simulink model "LAB3_Challenge_SSM_LQR_FS"  (R2020b)
settings: Solver=ode45  StartTime=0.0  StopTime=Time_of_simulation  RelTol=1e-3
undefined symbols (not defined in the file): Aq, Bb, Beq, Bq, daq, denH_w, DiscIntNeverNeededParam, drv, enable_integrator, gbox, Jb, Jh, K, K_I, Kaw, mld, mot, Nu, numH_w, Nxa, rads2rpm, sens, Step_ref, tausf, Ts
libraries: simulink x4
settings Model: Creator=Davide  LastModifiedBy=Musta

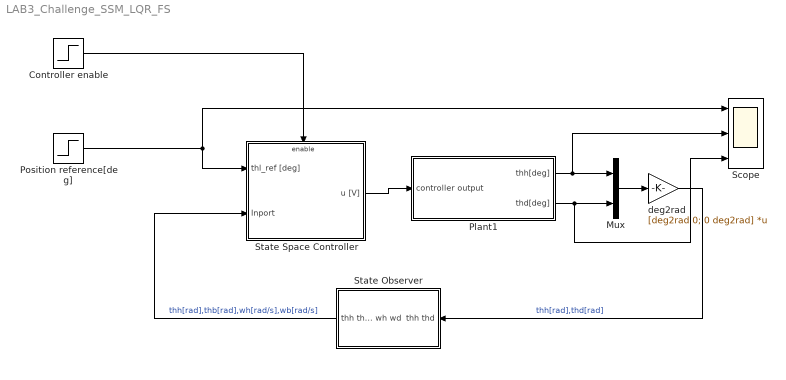
== system LAB3_Challenge_SSM_LQR_FS ==
  Controller enable : Step  Time=0.75  SampleTime=0
  Mux : Mux  Inputs=2
  Plant1 : Subsystem
  Position reference[deg] : Step  After=Step_ref  SampleTime=0
  Scope : Scope  NumInputPorts=3
  State Observer : Subsystem
  State Space Controller : Subsystem
  deg2rad : Gain  Gain=[deg2rad 0; 0 deg2rad]  Multiplication=Matrix(K*u) (u vector)
  wires:
  Position reference[deg]/1 -> Scope/1, State Space Controller/1(thl_ref [deg])
  Controller enable/1 -> State Space Controller/Enable
  Plant1/1(thh[deg]) -> Scope/2, Mux/1
  Mux/1 -> deg2rad/1
  deg2rad/1 -> State Observer/1(thh thd)  "thh[rad],thd[rad]"
  State Space Controller/1(u [V]) -> Plant1/1(controller output)
  Plant1/2(thd[deg]) -> Scope/3, Mux/2
  State Observer/1(thh thd wh wd) -> State Space Controller/2(Inport)  "thh[rad],thb[rad],wh[rad/s],wb[rad/s]"

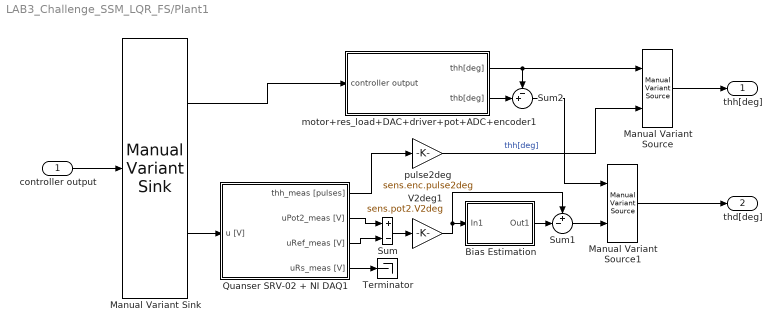
== system LAB3_Challenge_SSM_LQR_FS/Plant1 ==
  controller output : Inport
  Bias Estimation : Subsystem
  Manual Variant Sink : simulink/Signal Routing/Manual Variant Sink  NumChoices=2  LabelModeActiveChoice=V_2
  Manual Variant Source : simulink/Signal Routing/Manual Variant Source  NumChoices=2  LabelModeActiveChoice=V_2
  Manual Variant Source1 : simulink/Signal Routing/Manual Variant Source  NumChoices=2  LabelModeActiveChoice=V_2
  Quanser SRV-02 + NI DAQ1 : Subsystem  mask(Quanser SRV-02 (with resonant load) + NI DAQ){Ts=0.001, fricType=Karnopp, lockShaft=off, beamInitPos=10}
      mask prompts: Ts "NI DAQ Sample Time:"; fricType "Friction model"; lockShaft "Lock motor shaft"; beamInitPos "Beam initial position [deg]:"
      mask help: Quanser SRV-02 (with resonant load) + NI DAQ model.
      mask init:
      | %%
      | % Riccardo Antonello (riccardo.antonello@unipd.it)
      | %
      | % April 28, 2020
      | %
      | % Dept. of Information Engineering, University of Padova
      | %
      | 
      | %%  Conversion gains
      | deg2rad = pi/180;                   %   [deg]   -> [rad]
      | rad2deg = 180/pi;                   %   [rad]   -> [deg]
      | 
      | 
      | %%  Sensors data
      | 
      | %   shunt resistor
      | sens.curr.Rs = 0.5;   
      | 
      | %   Hewlett-Packard HEDS-5540#A06 optical encoder
      | sens.enc.ppr = 500*4;                                                   %   pulses per rotation
      | sens.enc.pulse2deg = 360/sens.enc.ppr;                                  %   [pulses] -> [deg]
      | sens.enc.pulse2rad = 2*pi/sens.enc.ppr;                                 %   [pulses] -> [rad]
      | sens.enc.deg2pulse = sens.enc.ppr/360;                                  %   [deg] -> [pulses]
      | sens.enc.rad2pulse = sens.enc.ppr/2/pi;                                 %   [rad] -> [pulses]
      | 
      | %   potentiometer 2 (Spectrol 357-0-0-103) - installed on hub
      | sens.pot2.range.R      = 10e3;                                          %   ohmic value range 
      | sens.pot2.range.V      = 5;                                             %   voltage range
      | sens.pot2.range.th_deg = 340;                                           %   angle range [deg]
      | sens.pot2.range.th     = sens.pot2.range.th_deg * deg2rad;              %   angle range [rad]                           
      | sens.pot2.deg2V        = sens.pot2.range.V / sens.pot2.range.th_deg;    %   sensitivity [V/deg]
      | sens.pot2.rad2V        = sens.pot2.range.V / sens.pot2.range.th;        %   sensitivity [V/rad]
      | sens.pot2.V2deg        = 1/sens.pot2.deg2V;                             %   conversion gain [V] -> [deg]
      | sens.pot2.V2rad        = 1/sens.pot2.rad2V;                             %   conversion gain [V] -> [rad]
      | sens.pot2.noise.var    = 3.5e-7;                                        %   out noise variance [V^2]
      | 
      | 
      | %%  Data acquisition board (daq) data
      | 
      | %   NI PCI-6221 DAC data
      | daq.dac.bits = 16;                                  %   resolution (bits)
      | daq.dac.fs   = 10;                                  %   full scale 
      | daq.dac.q    = 2*daq.dac.fs/(2^daq.dac.bits-1);     %	quantization
      | 
      | %   NI PCI-6221 ADC data
      | daq.adc.bits = 16;                                  %   resolution (bits)
      | daq.adc.fs   = 10;                                  %   full scale (as set in SLDRT Analog Input block)
      | daq.adc.q    = 2*daq.adc.fs/(2^daq.adc.bits-1);     %   quantization   
      | 
      | 
      | %%  Set beam initial position
      | % SRV02Handle = find_system(gcb, ...
      | %     'LookUnderMasks', 'on', ...
      | %     'FindAll', 'on', ...
      | %     'FollowLinks', 'on', ...
      | %     'SearchDepth', '1', ...
      | %     'BlockType', 'ModelReference', ...
      | %     'Name', 'Quanser SRV-02');
      | %
      | % %get_param(SRV02Handle, 'InstanceParameters')
      | % InstanceParams = get_param(SRV02Handle, 'InstanceParameters');
      | % for k = 1:length(InstanceParams)
      | %     if strcmp(InstanceParams(k).Name, 'thb0')
      | %         if lockShaft
      | %             InstanceParams(k).Value = sprintf('%f', beamInitPos);
      | %         else
      | %             InstanceParams(k).Value = sprintf('%f', 0);    
      | %         end
      | %         set_param(SRV02Handle, 'InstanceParameters', InstanceParams);
      | %         break;
      | %     end
      | % end
      | 
      | if lockShaft
      |     thb0 = beamInitPos;
      | else
      |     thb0 = 0;    
      | end
      | 
      | 
      | %%  Mask initialization
      | if lockShaft
      |     
      |     %   find Inport handle
      |     InPortHandle = find_system(gcb, ...
      |         'LookUnderMasks', 'on', ...
      |         'FindAll', 'on', ...
      |         'FollowLinks', 'on', ...
      |         'SearchDepth', '1', ...
      |         'BlockType', 'Inport', ...
      |         'Name', 'u [V]');
      |     
      |     if ~isempty(InPortHandle)
      |     
      |         %   find DAC handle
      |         DACHandle = find_system(gcb, ...
      |             'LookUnderMasks', 'on', ...
      |             'FindAll', 'on', ...
      |             'FollowLinks', 'on', ...
      |             'SearchDepth', '1', ...
      |             'BlockType', 'SubSystem', ...
      |             'Name', 'DAC');  
      | 
      |         %   remove Inport output connection   
      |         InportConn = get_param(InPortHandle, 'PortConnectivity');
      |         delete_line(gcb, InportConn.Position);
      | 
      |         %   remove Inport block
      |         delete_block(InPortHandle);
      | 
      |         %   add Constant block
      |         ConstantHandle = add_block( ...
      |             'simulink/Sources/Constant', [gcb, '/u [V]'], ...
      |             'Position', [20   -37    50   -23], ...
      |             'Value', '0');
      | 
      |         %   connect Constant to DAC block
      |         DACPortHandles = get_param(DACHandle, 'PortHandles');
      |         ConstantPortHandles = get_param(ConstantHandle, 'PortHandles');
      |         add_line(gcb, ConstantPortHandles.Outport(1), DACPortHandles.Inport(1));
      |     
      |     end
      |     
      | else
      |     
      |     %   find Constant handle
      |     ConstantHandle = find_system(gcb, ...
      |         'LookUnderMasks', 'on', ...
      |         'FindAll', 'on', ...
      |         'FollowLinks', 'on', ...
      |         'SearchDepth', '1', ...
      |         'BlockType', 'Constant', ...
      |         'Name', 'u [V]');
      |     
      |     if ~isempty(ConstantHandle)
      |     
      |         %   find DAC handle
      |         DACHandle = find_system(gcb, ...
      |             'LookUnderMasks', 'on', ...
      |             'FindAll', 'on', ...
      |             'FollowLinks', 'on', ...
      |             'SearchDepth', '1', ...
      |             'BlockType', 'SubSystem', ...
      |             'Name', 'DAC');  
      |  
      |         %   remove Constant output connection   
      |         ConstantConn = get_param(ConstantHandle, 'PortConnectivity');
      |         delete_line(gcb, ConstantConn.Position);
      | 
      |         %   remove Inport block
      |         delete_block(ConstantHandle);   
      | 
      |         %   add Inport block
      |         InportHandle = add_block( ...
      |             'simulink/Sources/In1', [gcb, '/u [V]'], ...
      |             'Position', [20   -37    50   -23], ...
      |             'Port', '1');
      | 
      |         %   connect Constant to DAC block
      |         DACPortHandles = get_param(DACHandle, 'PortHandles');
      |         InportPortHandles = get_param(InportHandle, 'PortHandles');
      |         add_line(gcb, InportPortHandles.Outport(1), DACPortHandles.Inport(1));
      |     
      |      end
      |     
      | end
      mask Help:
      | Riccardo Antonello (antonello@dei.unipd.it)
      | 
      | April 28, 2020
      | 
      | Dept. of Information Engineering, University of Padova
      mask TypeOptions fricType: Coulomb + viscous | Karnopp
      mask Callback lockShaft:
      | %   get status of check box
      | lockShaft = get_param(gcb, 'lockShaft');
      | 
      | %   get current value of MaskVisibilities property
      | maskVisibilities = get_param(gcb, 'MaskVisibilities');
      | 
      | %   set visibility of the dialog box element
      | if strcmp(lockShaft, 'on')
      |     maskVisibilities{4} = 'on';
      | else
      |     maskVisibilities{4} = 'off';
      | end
      | 
      | % Set the 'MaskVisibilities' property for each parameter in mask
      | set_param( gcb, 'MaskVisibilities', maskVisibilities);
  Sum : Sum  Inputs=+-
  Sum1 : Sum  Inputs=+-|
  Sum2 : Sum  Inputs=-+|
  Terminator : Terminator
  V2deg1 : Gain  Gain=sens.pot2.V2deg
  motor+res_load+DAC+driver+pot+ADC+encoder1 : Subsystem
  pulse2deg : Gain  Gain=sens.enc.pulse2deg
  thh[deg] : Outport
  thd[deg] : Outport  Port=2
  wires:
  V2deg1/1 -> Bias Estimation/1(In1), Sum1/1
  Quanser SRV-02 + NI DAQ1/2(uPot2_meas [V]) -> Sum/1
  Sum/1 -> V2deg1/1
  Quanser SRV-02 + NI DAQ1/3(uRef_meas [V]) -> Sum/2
  pulse2deg/1 -> Manual Variant Source/2  "thh[deg]"
  Sum2/1 -> Manual Variant Source1/1
  motor+res_load+DAC+driver+pot+ADC+encoder1/2(thb[deg]) -> Sum2/2
  Sum1/1 -> Manual Variant Source1/2
  Bias Estimation/1(Out1) -> Sum1/2
  Quanser SRV-02 + NI DAQ1/1(thh_meas [pulses]) -> pulse2deg/1
  Manual Variant Source/1 -> thh[deg]/1
  motor+res_load+DAC+driver+pot+ADC+encoder1/1(thh[deg]) -> Manual Variant Source/1, Sum2/1
  Manual Variant Sink/2 -> Quanser SRV-02 + NI DAQ1/1(u [V])
  Manual Variant Sink/1 -> motor+res_load+DAC+driver+pot+ADC+encoder1/1(controller output)
  controller output/1 -> Manual Variant Sink/1
  Manual Variant Source1/1 -> thd[deg]/1
  Quanser SRV-02 + NI DAQ1/4(uRs_meas [V]) -> Terminator/1

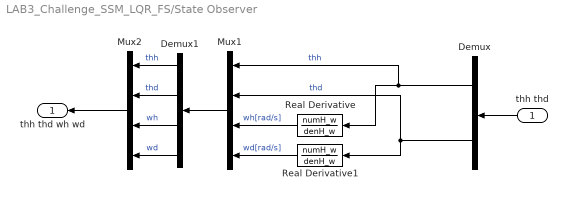
== system LAB3_Challenge_SSM_LQR_FS/State Observer ==
  thh thd : Inport
  Demux : Demux  Outputs=2
  Demux1 : Demux
  Mux1 : Mux
  Mux2 : Mux
  Real Derivative : TransferFcn  Numerator=numH_w  Denominator=denH_w
  Real Derivative1 : TransferFcn  Numerator=numH_w  Denominator=denH_w
  thh thd wh wd : Outport
  wires:
  Real Derivative/1 -> Mux1/3  "wh[rad/s]"
  Demux/1 -> Real Derivative/1, Mux1/1  "thh"
  thh thd/1 -> Demux/1
  Real Derivative1/1 -> Mux1/4  "wd[rad/s]"
  Demux/2 -> Mux1/2, Real Derivative1/1  "thd"
  Mux2/1 -> thh thd wh wd/1
  Mux1/1 -> Demux1/1
  Demux1/1 -> Mux2/1  "thh"
  Demux1/2 -> Mux2/2  "thd"
  Demux1/3 -> Mux2/3  "wh"
  Demux1/4 -> Mux2/4  "wd"

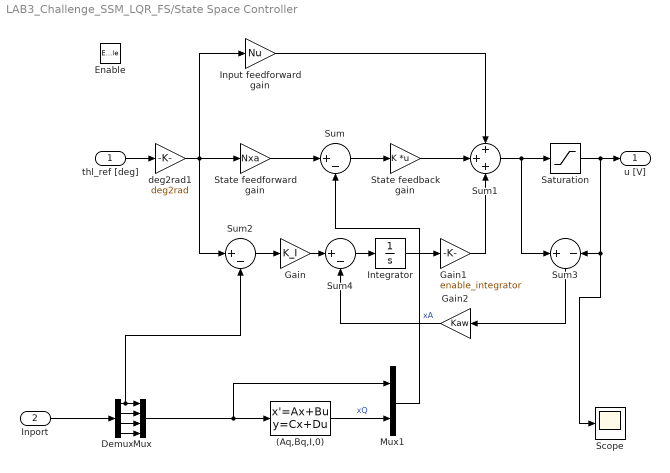
== system LAB3_Challenge_SSM_LQR_FS/State Space Controller ==
  thl_ref [deg] : Inport
  Inport : Inport  Port=2
  Enable : EnablePort
  (Aq,Bq,I,0) : StateSpace  A=Aq  B=Bq  C=eye(2)  D=zeros(2,4)  InitialCondition=0
  Demux : Demux
  Gain : Gain  Gain=K_I
  Gain1 : Gain  Gain=enable_integrator
  Gain2 : Gain  Gain=Kaw
  Input feedforward gain : Gain  Gain=Nu
  Integrator : Integrator
  Mux : Mux
  Mux1 : Mux  Inputs=2
  Saturation : Saturate  UpperLimit=daq.dac.fs  LowerLimit=-daq.dac.fs
  Scope : Scope
  State feedback gain : Gain  Gain=K  Multiplication=Matrix(K*u)
  State feedforward gain : Gain  Gain=Nxa
  Sum : Sum  Inputs=|+-
  Sum1 : Sum  Inputs=+++
  Sum2 : Sum  Inputs=|+-
  Sum3 : Sum  Inputs=+|-
  Sum4 : Sum  Inputs=|+-
  deg2rad1 : Gain  Gain=deg2rad
  u [V] : Outport
  wires:
  Sum1/1 -> Sum3/1, Saturation/1
  Saturation/1 -> Scope/1, Sum3/2, u [V]/1
  Mux1/1 -> Sum/2  "xA"
  thl_ref [deg]/1 -> deg2rad1/1
  deg2rad1/1 -> Sum2/1, State feedforward gain/1, Input feedforward gain/1
  Input feedforward gain/1 -> Sum1/1
  State feedforward gain/1 -> Sum/1
  Sum/1 -> State feedback gain/1
  State feedback gain/1 -> Sum1/2
  (Aq,Bq,I,0)/1 -> Mux1/2  "xQ"
  Sum2/1 -> Gain/1
  Gain/1 -> Sum4/1
  Integrator/1 -> Gain1/1
  Gain1/1 -> Sum1/3
  Sum4/1 -> Integrator/1
  Gain2/1 -> Sum4/2
  Sum3/1 -> Gain2/1
  Demux/4 -> Mux/4
  Demux/1 -> Sum2/2, Mux/1
  Demux/2 -> Mux/2
  Demux/3 -> Mux/3
  Inport/1 -> Demux/1
  Mux/1 -> Mux1/1, (Aq,Bq,I,0)/1

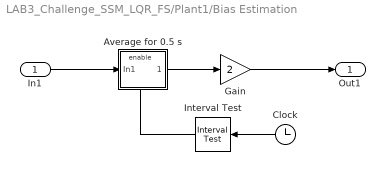
== system LAB3_Challenge_SSM_LQR_FS/Plant1/Bias Estimation ==
  In1 : Inport
  Average for 0.5 s : Subsystem
  Clock : Clock
  Gain : Gain  Gain=2
  Interval Test : simulink/Logic and Bit Operations/Interval Test  IntervalClosedRight=on  uplimit=0.7  IntervalClosedLeft=on  lowlimit=0.2  OutDataTypeStr=boolean
  Out1 : Outport
  wires:
  Interval Test/1 -> Average for 0.5 s/Enable
  In1/1 -> Average for 0.5 s/1(In1)
  Clock/1 -> Interval Test/1
  Average for 0.5 s/1(Out1) -> Gain/1
  Gain/1 -> Out1/1

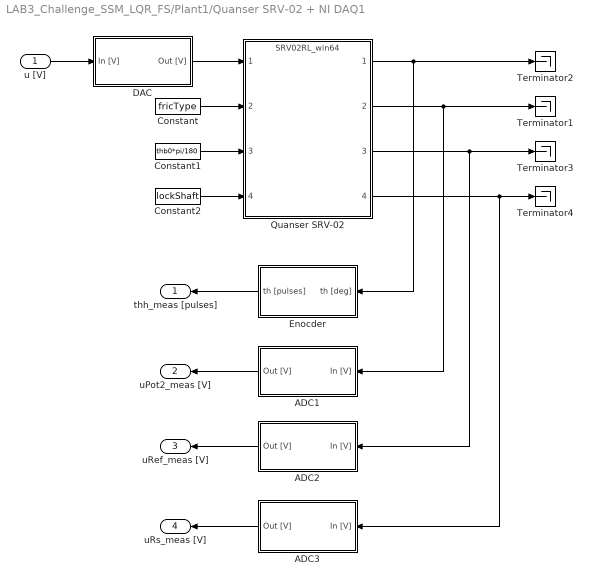
== system LAB3_Challenge_SSM_LQR_FS/Plant1/Quanser SRV-02 + NI DAQ1 ==
  u [V] : Inport
  ADC1 : Subsystem
  ADC2 : Subsystem
  ADC3 : Subsystem
  Constant : Constant  Value=fricType
  Constant1 : Constant  Value=thb0*pi/180  SampleTime=Inf
  Constant2 : Constant  Value=lockShaft  SampleTime=Inf
  DAC : Subsystem
  Enocder : Subsystem
  Quanser SRV-02 : ModelReference  ModelNameDialog=SRV02RL_win64.slxp  ModelReferenceVersion=1.76  CopyOfModelProtected=on
  Terminator{1..4} (4 alike) : Terminator
  thh_meas [pulses] : Outport
  uPot2_meas [V] : Outport  Port=2
  uRef_meas [V] : Outport  Port=3
  uRs_meas [V] : Outport  Port=4
  wires:
  Enocder/1(th [pulses]) -> thh_meas [pulses]/1
  ADC3/1(Out [V]) -> uRs_meas [V]/1
  DAC/1(Out [V]) -> Quanser SRV-02/1
  Quanser SRV-02/2 -> ADC1/1(In [V]), Terminator1/1
  Quanser SRV-02/1 -> Terminator2/1, Enocder/1(th [deg])
  Constant/1 -> Quanser SRV-02/2
  Quanser SRV-02/3 -> ADC2/1(In [V]), Terminator3/1
  ADC1/1(Out [V]) -> uPot2_meas [V]/1
  Constant1/1 -> Quanser SRV-02/3
  Constant2/1 -> Quanser SRV-02/4
  Quanser SRV-02/4 -> ADC3/1(In [V]), Terminator4/1
  ADC2/1(Out [V]) -> uRef_meas [V]/1
  u [V]/1 -> DAC/1(In [V])

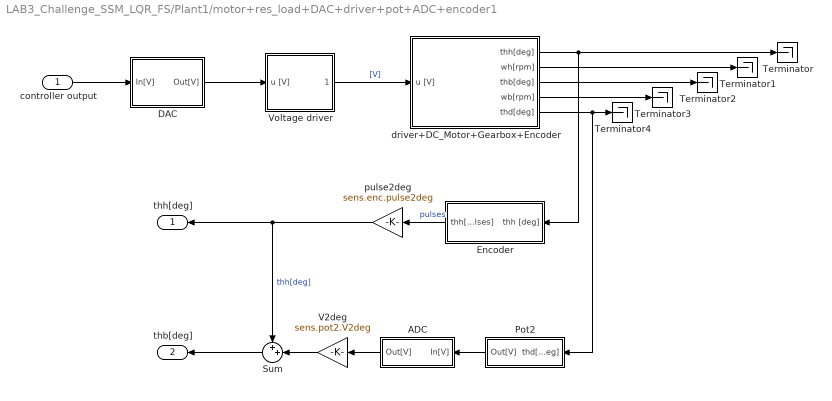
== system LAB3_Challenge_SSM_LQR_FS/Plant1/motor+res_load+DAC+driver+pot+ADC+encoder1 ==
  controller output : Inport
  ADC : Subsystem
  DAC : Subsystem
  Encoder : Subsystem
  Pot2 : Subsystem
  Sum : Sum  Inputs=++|
  Terminator{,1..4} (5 alike) : Terminator
  V2deg : Gain  Gain=sens.pot2.V2deg
  Voltage driver : Subsystem
  driver+DC_Motor+Gearbox+Encoder : Subsystem
  pulse2deg : Gain  Gain=sens.enc.pulse2deg
  thh[deg] : Outport
  thb[deg] : Outport  Port=2
  wires:
  Encoder/1(thh[pulses]) -> pulse2deg/1  "pulses"
  Sum/1 -> thb[deg]/1
  Pot2/1(Out[V]) -> ADC/1(In[V])
  driver+DC_Motor+Gearbox+Encoder/5(thd[deg]) -> Terminator4/1, Pot2/1(thd[deg])
  driver+DC_Motor+Gearbox+Encoder/1(thh[deg]) -> Terminator/1, Encoder/1("thh [deg] ")
  driver+DC_Motor+Gearbox+Encoder/3(thb[deg]) -> Terminator2/1
  controller output/1 -> DAC/1(In[V])
  DAC/1(Out[V]) -> Voltage driver/1(u [V])
  V2deg/1 -> Sum/2
  ADC/1(Out[V]) -> V2deg/1
  driver+DC_Motor+Gearbox+Encoder/2(wh[rpm]) -> Terminator1/1
  pulse2deg/1 -> thh[deg]/1, Sum/1  "thh[deg]"
  Voltage driver/1(udrv [V]) -> driver+DC_Motor+Gearbox+Encoder/1(u [V])  "[V]"
  driver+DC_Motor+Gearbox+Encoder/4(wb[rpm]) -> Terminator3/1

== system LAB3_Challenge_SSM_LQR_FS/Plant1/Bias Estimation/Average for 0.5 s ==
  In1 : Inport
  Enable : EnablePort
  Discrete-Time Integrator : DiscreteIntegrator  SampleTime=Ts  ICPrevOutput=DiscIntNeverNeededParam  ICPrevScaledInput=DiscIntNeverNeededParam
  Out1 : Outport
  wires:
  In1/1 -> Discrete-Time Integrator/1
  Discrete-Time Integrator/1 -> Out1/1

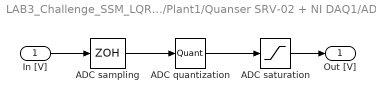
== system LAB3_Challenge_SSM_LQR_FS/Plant1/Quanser SRV-02 + NI DAQ1/ADC1 ==
  In [V] : Inport
  ADC quantization : Quantizer  QuantizationInterval=daq.adc.q
  ADC sampling : ZeroOrderHold  SampleTime=Ts
  ADC saturation : Saturate  UpperLimit=daq.adc.fs  LowerLimit=-daq.adc.fs
  Out [V] : Outport
  wires:
  ADC saturation/1 -> Out [V]/1
  ADC sampling/1 -> ADC quantization/1
  In [V]/1 -> ADC sampling/1
  ADC quantization/1 -> ADC saturation/1

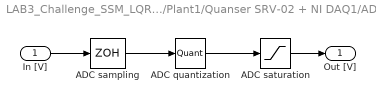
== system LAB3_Challenge_SSM_LQR_FS/Plant1/Quanser SRV-02 + NI DAQ1/ADC2 ==
  In [V] : Inport
  ADC quantization : Quantizer  QuantizationInterval=daq.adc.q
  ADC sampling : ZeroOrderHold  SampleTime=Ts
  ADC saturation : Saturate  UpperLimit=daq.adc.fs  LowerLimit=-daq.adc.fs
  Out [V] : Outport
  wires:
  ADC quantization/1 -> ADC saturation/1
  In [V]/1 -> ADC sampling/1
  ADC sampling/1 -> ADC quantization/1
  ADC saturation/1 -> Out [V]/1

== system LAB3_Challenge_SSM_LQR_FS/Plant1/Quanser SRV-02 + NI DAQ1/ADC3 ==
  In [V] : Inport
  Quantizer : Quantizer  QuantizationInterval=daq.adc.q
  Saturation : Saturate  UpperLimit=daq.adc.fs  LowerLimit=-daq.adc.fs
  Zero-Order Hold : ZeroOrderHold  SampleTime=Ts
  Out [V] : Outport
  wires:
  Saturation/1 -> Out [V]/1
  In [V]/1 -> Zero-Order Hold/1
  Quantizer/1 -> Saturation/1
  Zero-Order Hold/1 -> Quantizer/1

== system LAB3_Challenge_SSM_LQR_FS/Plant1/Quanser SRV-02 + NI DAQ1/DAC ==
  In [V] : Inport
  Quantizer : Quantizer  QuantizationInterval=daq.dac.q
  Saturation : Saturate  UpperLimit=daq.dac.fs  LowerLimit=-daq.dac.fs
  Zero-Order Hold : ZeroOrderHold  SampleTime=Ts
  Out [V] : Outport
  wires:
  Quantizer/1 -> Saturation/1
  In [V]/1 -> Zero-Order Hold/1
  Zero-Order Hold/1 -> Quantizer/1
  Saturation/1 -> Out [V]/1

== system LAB3_Challenge_SSM_LQR_FS/Plant1/Quanser SRV-02 + NI DAQ1/Enocder ==
  th [deg] : Inport
  Quantizer : Quantizer  QuantizationInterval=sens.enc.pulse2deg
  Zero-Order Hold : ZeroOrderHold  SampleTime=Ts
  deg2pulse : Gain  Gain=sens.enc.deg2pulse
  th [pulses] : Outport
  wires:
  Quantizer/1 -> deg2pulse/1
  th [deg]/1 -> Zero-Order Hold/1
  Zero-Order Hold/1 -> Quantizer/1
  deg2pulse/1 -> th [pulses]/1

== system LAB3_Challenge_SSM_LQR_FS/Plant1/motor+res_load+DAC+driver+pot+ADC+encoder1/ADC ==
  In[V] : Inport
  ADC quantization : Quantizer  QuantizationInterval=daq.adc.q
  ADC sampling : ZeroOrderHold  SampleTime=Ts
  ADC saturation : Saturate  UpperLimit=daq.adc.fs  LowerLimit=-daq.adc.fs
  Out[V] : Outport
  wires:
  ADC quantization/1 -> ADC saturation/1
  In[V]/1 -> ADC sampling/1
  ADC sampling/1 -> ADC quantization/1
  ADC saturation/1 -> Out[V]/1

== system LAB3_Challenge_SSM_LQR_FS/Plant1/motor+res_load+DAC+driver+pot+ADC+encoder1/DAC ==
  In[V] : Inport
  Quantizer : Quantizer  QuantizationInterval=daq.dac.q
  Saturation : Saturate  UpperLimit=daq.dac.fs  LowerLimit=-daq.dac.fs  LinearizeAsGain=off
  Zero-Order Hold : ZeroOrderHold  SampleTime=Ts
  Out[V] : Outport
  wires:
  Saturation/1 -> Out[V]/1
  Zero-Order Hold/1 -> Quantizer/1
  Quantizer/1 -> Saturation/1
  In[V]/1 -> Zero-Order Hold/1

== system LAB3_Challenge_SSM_LQR_FS/Plant1/motor+res_load+DAC+driver+pot+ADC+encoder1/Encoder ==
  "thh [deg] " : Inport
  Gain : Gain  Gain=sens.enc.ppr/360
  Quantizer : Quantizer  QuantizationInterval=sens.enc.pulse2deg
  Zero-Order Hold : ZeroOrderHold  SampleTime=Ts
  thh[pulses] : Outport
  wires:
  Gain/1 -> thh[pulses]/1
  Quantizer/1 -> Gain/1
  Zero-Order Hold/1 -> Quantizer/1
  "thh [deg] "/1 -> Zero-Order Hold/1

== system LAB3_Challenge_SSM_LQR_FS/Plant1/motor+res_load+DAC+driver+pot+ADC+encoder1/Pot2 ==
  thd[deg] : Inport
  Sensor Output Noise [V] : RandomNumber  Variance=sens.pot2.noise.var  SampleTime=Ts
  Sum : Sum  Inputs=|++
  deg2V : Gain  Gain=sens.pot2.deg2V
  Out[V] : Outport
  wires:
  thd[deg]/1 -> deg2V/1
  deg2V/1 -> Sum/1
  Sensor Output Noise [V]/1 -> Sum/2
  Sum/1 -> Out[V]/1

== system LAB3_Challenge_SSM_LQR_FS/Plant1/motor+res_load+DAC+driver+pot+ADC+encoder1/Voltage driver ==
  u [V] : Inport
  Saturation : Saturate  UpperLimit=drv.outmax  LowerLimit=-drv.outmax  LinearizeAsGain=off
  Transfer Fcn : TransferFcn  Numerator=[drv.dcgain]  Denominator=[drv.Tc 1]
  udrv [V] : Outport
  wires:
  Saturation/1 -> udrv [V]/1
  Transfer Fcn/1 -> Saturation/1
  u [V]/1 -> Transfer Fcn/1

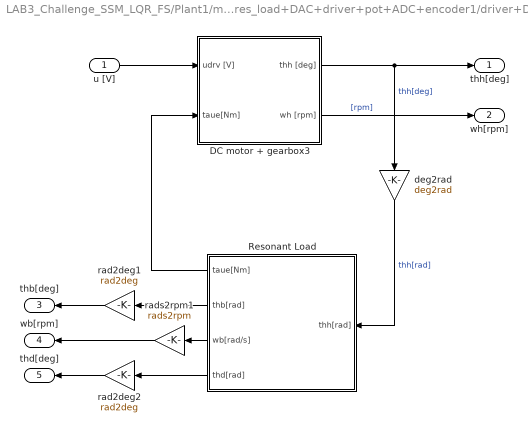
== system LAB3_Challenge_SSM_LQR_FS/Plant1/motor+res_load+DAC+driver+pot+ADC+encoder1/driver+DC_Motor+Gearbox+Encoder ==
  u [V] : Inport
  DC motor + gearbox3 : Subsystem
  Resonant Load : Subsystem
  deg2rad : Gain  Gain=deg2rad
  rad2deg1 : Gain  Gain=rad2deg
  rad2deg2 : Gain  Gain=rad2deg
  rads2rpm1 : Gain  Gain=rads2rpm
  thh[deg] : Outport
  wh[rpm] : Outport  Port=2
  thb[deg] : Outport  Port=3
  wb[rpm] : Outport  Port=4
  thd[deg] : Outport  Port=5
  wires:
  DC motor + gearbox3/2(wh [rpm]) -> wh[rpm]/1  "[rpm]"
  DC motor + gearbox3/1("thh [deg] ") -> thh[deg]/1, deg2rad/1  "thh[deg]"
  u [V]/1 -> DC motor + gearbox3/1(udrv [V])
  deg2rad/1 -> Resonant Load/1(thh[rad])  "thh[rad]"
  Resonant Load/1(taue[Nm]) -> DC motor + gearbox3/2(taue[Nm])
  Resonant Load/2(thb[rad]) -> rad2deg1/1
  Resonant Load/3(wb[rad/s]) -> rads2rpm1/1
  Resonant Load/4(thd[rad]) -> rad2deg2/1
  rad2deg1/1 -> thb[deg]/1
  rads2rpm1/1 -> wb[rpm]/1
  rad2deg2/1 -> thd[deg]/1

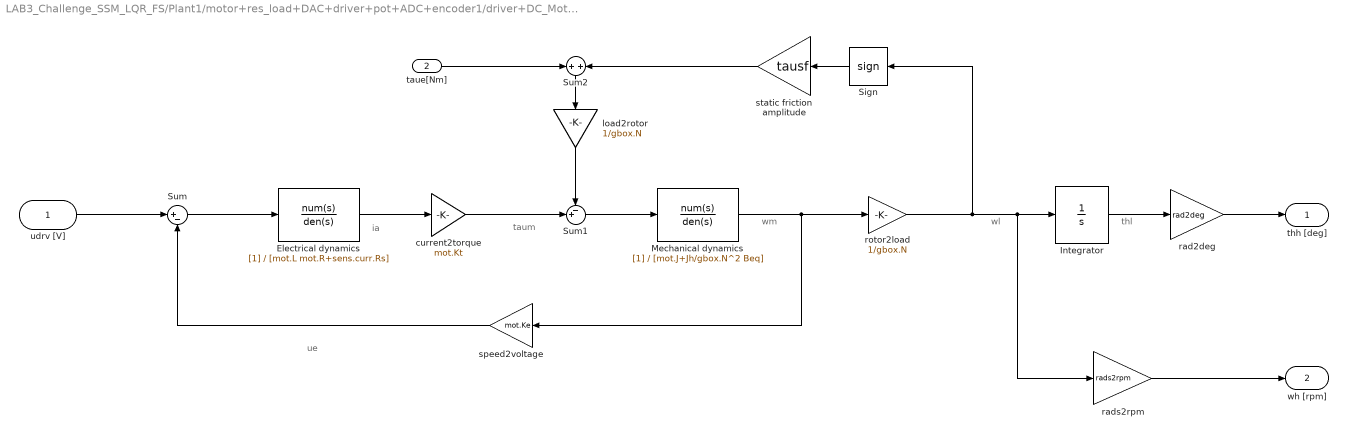
== system LAB3_Challenge_SSM_LQR_FS/Plant1/motor+res_load+DAC+driver+pot+ADC+encoder1/driver+DC_Motor+Gearbox+Encoder/DC motor + gearbox3 ==
  note: thl
  note: wl
  note: wm
  note: ue
  note: taum
  note: ia
  udrv [V] : Inport
  taue[Nm] : Inport  Port=2
  Electrical dynamics : TransferFcn  Denominator=[mot.L mot.R+sens.curr.Rs]
  Integrator : Integrator
  Mechanical dynamics : TransferFcn  Denominator=[mot.J+Jh/gbox.N^2 Beq]
  Sign : Signum  ZeroCross=off
  Sum : Sum  Inputs=|+-
  Sum1 : Sum  Inputs=-+|
  Sum2 : Sum  Inputs=+|+
  current2torque : Gain  Gain=mot.Kt
  load2rotor : Gain  Gain=1/gbox.N
  rad2deg : Gain  Gain=rad2deg
  rads2rpm : Gain  Gain=rads2rpm
  rotor2load : Gain  Gain=1/gbox.N
  speed2voltage : Gain  Gain=mot.Ke
  static friction amplitude : Gain  Gain=tausf
  "thh [deg] " : Outport
  wh [rpm] : Outport  Port=2
  wires:
  udrv [V]/1 -> Sum/1
  Electrical dynamics/1 -> current2torque/1
  Sign/1 -> static friction amplitude/1
  speed2voltage/1 -> Sum/2
  rad2deg/1 -> "thh [deg] "/1
  Mechanical dynamics/1 -> speed2voltage/1, rotor2load/1
  rads2rpm/1 -> wh [rpm]/1
  Sum/1 -> Electrical dynamics/1
  rotor2load/1 -> Sign/1, rads2rpm/1, Integrator/1
  Integrator/1 -> rad2deg/1
  Sum1/1 -> Mechanical dynamics/1
  load2rotor/1 -> Sum1/1
  current2torque/1 -> Sum1/2
  Sum2/1 -> load2rotor/1
  static friction amplitude/1 -> Sum2/2
  taue[Nm]/1 -> Sum2/1

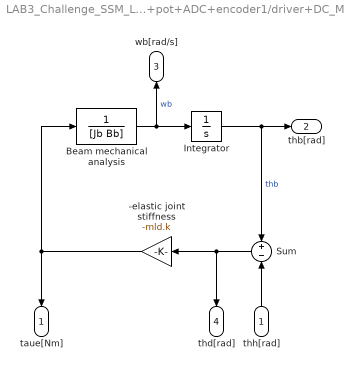
== system LAB3_Challenge_SSM_LQR_FS/Plant1/motor+res_load+DAC+driver+pot+ADC+encoder1/driver+DC_Motor+Gearbox+Encoder/Resonant Load ==
  thh[rad] : Inport
  -elastic joint stiffness : Gain  Gain=-mld.k
  Beam mechanical analysis : TransferFcn  Denominator=[Jb Bb]
  Integrator : Integrator
  Sum : Sum  Inputs=+|-
  taue[Nm] : Outport
  thb[rad] : Outport  Port=2
  wb[rad/s] : Outport  Port=3
  thd[rad] : Outport  Port=4
  wires:
  Sum/1 -> -elastic joint stiffness/1, thd[rad]/1
  Integrator/1 -> thb[rad]/1, Sum/1  "thb"
  -elastic joint stiffness/1 -> Beam mechanical analysis/1, taue[Nm]/1
  thh[rad]/1 -> Sum/2
  Beam mechanical analysis/1 -> Integrator/1, wb[rad/s]/1  "wb"
